simulink model "hydrod"  (Simulink 6.0)
settings: Solver=ode45  SolverMode=SingleTasking  StartTime=0.0  StopTime=0.1  RelTol=1e-3  AbsTol=1e-6
PreLoadFcn:
  | load newhcd
undefined symbols (not defined in the file or in its folder): Ac, C2, I, L, M, Qmax
libraries: hydlib x4, simulink x2
settings Model: CovMetricSettings=d  Creator=The MathWorks Inc.  LastModifiedBy=batserve  ExtModeTrigMode=oneshot  ExtModeArmWhenConnect=off  ExtModeAutoUpdateStatusClock=off
settings DataIOCC: LimitDataPoints=off  SaveOutput=off  SaveState=on
settings OptimizationCC: BlockReduction=off  BooleanDataType=off
settings DebuggingCC: AlgebraicLoopMsg=none  CheckExecutionContextPreStartOutputMsg=on  CheckExecutionContextRuntimeOutputMsg=on  SolverPrmCheckMsg=none  IntegerOverflowMsg=none
settings HardwareCC: TargetUnknown=on

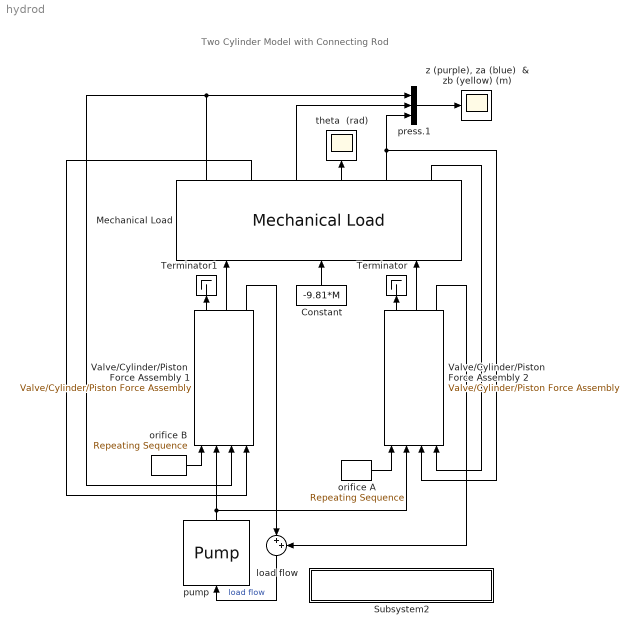
== system hydrod ==
  note: Two Cylinder Model with Connecting Rod
  Constant : Constant  Orientation=up  Value=-9.81*M
  Mechanical Load : hydlib/Mechanical Load  Orientation=up  L=L  M=M  I=I
  Subsystem2 : Subsystem  PropExecContextAcrossSSBoundary=on
      settings: OpenFcn=sim(get_param(0, 'CurrentSystem'), 0.1)
      mask Type: Button
      mask Display: disp('Double click to run the\nSimulation for 0.1 seconds')
  Terminator : Terminator
      settings: Orientation=up
  Terminator1 : Terminator
      settings: Orientation=up
  Valve/Cylinder/Piston  Force Assembly 1 : hydlib/Valve//Cylinder//Piston Force Assembly  Orientation=up  C1=C1  Ac=Ac  Cd=Cd  rho=rho  V30=V30  beta=Beta  p30=9.81*M/2/Ac
  Valve/Cylinder/Piston  Force Assembly 2 : hydlib/Valve//Cylinder//Piston Force Assembly  Orientation=up  C1=C1  Ac=Ac  Cd=Cd  rho=rho  V30=V30  beta=Beta  p30=9.81*M/2/Ac
  load flow : Sum  Orientation=down  Inputs=|++  SaturateOnIntegerOverflow=on  InputSameDT=on
  orifice A : simulink/Sources/Repeating Sequence  rep_seq_t="[0  0.1  0.2]/10"  rep_seq_y=[1 0 1]*1e-5
  orifice B : simulink/Sources/Repeating Sequence  rep_seq_t=[0 0.1 0.2]/10  rep_seq_y=[0 1 0]*1e-5
  press.1 : Mux  Inputs=3
  pump : hydlib/Pump  Orientation=up  t="[0        .04]"  Qpump=Qmax*[1 1]  p10=9.81*M/2/Ac  C2=C2/10
  theta  (rad) : Scope
      settings: Orientation=up  TickLabels=on  TimeRange=0.1  YMin=-0.0015  YMax=0.0005  DataFormat=Array
  "z (purple), za (blue)  & zb (yellow) (m)" : Scope
      settings: TickLabels=on  TimeRange=0.1  YMin=-0.005  YMax=0.015  DataFormat=Array
  wires:
  Mechanical Load/1 -> press.1/1, Valve/Cylinder/Piston  Force Assembly 1/3
  Mechanical Load/5 -> press.1/3, Valve/Cylinder/Piston  Force Assembly 2/3
  Mechanical Load/3 -> press.1/2
  Mechanical Load/4 -> theta  (rad)/1
  Constant/1 -> Mechanical Load/2
  press.1/1 -> "z (purple), za (blue)  & zb (yellow) (m)"/1
  Valve/Cylinder/Piston  Force Assembly 2/2 -> Mechanical Load/3
  Mechanical Load/6 -> Valve/Cylinder/Piston  Force Assembly 2/4
  orifice A/1 -> Valve/Cylinder/Piston  Force Assembly 2/1
  Valve/Cylinder/Piston  Force Assembly 2/1 -> Terminator/1
  Valve/Cylinder/Piston  Force Assembly 1/2 -> Mechanical Load/1
  Mechanical Load/2 -> Valve/Cylinder/Piston  Force Assembly 1/4
  orifice B/1 -> Valve/Cylinder/Piston  Force Assembly 1/1
  Valve/Cylinder/Piston  Force Assembly 1/1 -> Terminator1/1
  pump/1 -> Valve/Cylinder/Piston  Force Assembly 1/2, Valve/Cylinder/Piston  Force Assembly 2/2
  load flow/1 -> pump/1  "load flow"
  Valve/Cylinder/Piston  Force Assembly 2/3 -> load flow/2
  Valve/Cylinder/Piston  Force Assembly 1/3 -> load flow/1

== system hydrod/Subsystem2 ==
